simulink model "PID2"  (R2022b)
settings: Solver=VariableStepAuto  StartTime=0.0  StopTime=20  RelTol=1e-3
values from neighbouring files (symbols this model uses):
  g = 9.8    [config.m]
  Jx = 2*Mc*R^2/5 + 2*m*l^2    (= 0.0448)    [config.m]
  Jy = 2*Mc*R^2/5 + 2*m*l^2    (= 0.0448)    [config.m]
  Jz = 2*Mc*R^2/5 + 4*m*l^2    (= 0.0808)    [config.m]
  Kd_pitch = 15    [config.m]
  Kd_roll = 15    [config.m]
  Kd_yaw = 15    [config.m]
  Kd_z = 15    [config.m]
  Ki_pitch = 1    [config.m]
  Ki_roll = 1    [config.m]
  Ki_yaw = 1    [config.m]
  Ki_z = 10    [config.m]
  Kp_pitch = 80    [config.m]
  Kp_roll = 80    [config.m]
  Kp_yaw = 80    [config.m]
  Kp_z = 80    [config.m]
  M = Mc + 4*m    (= 3)    [config.m]
settings Model: Creator=cxk  LastModifiedBy=cxk

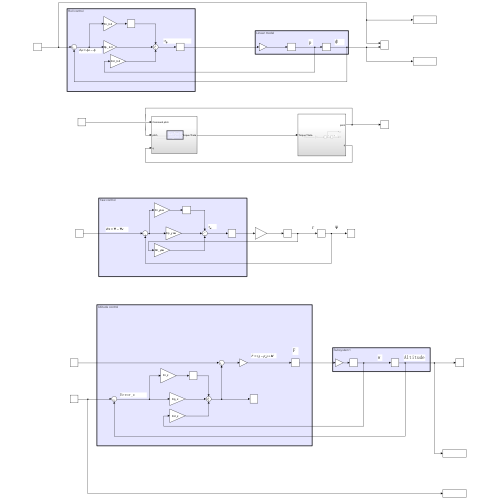
[thumbnail: Simulink's stored preview of the top-level diagram]
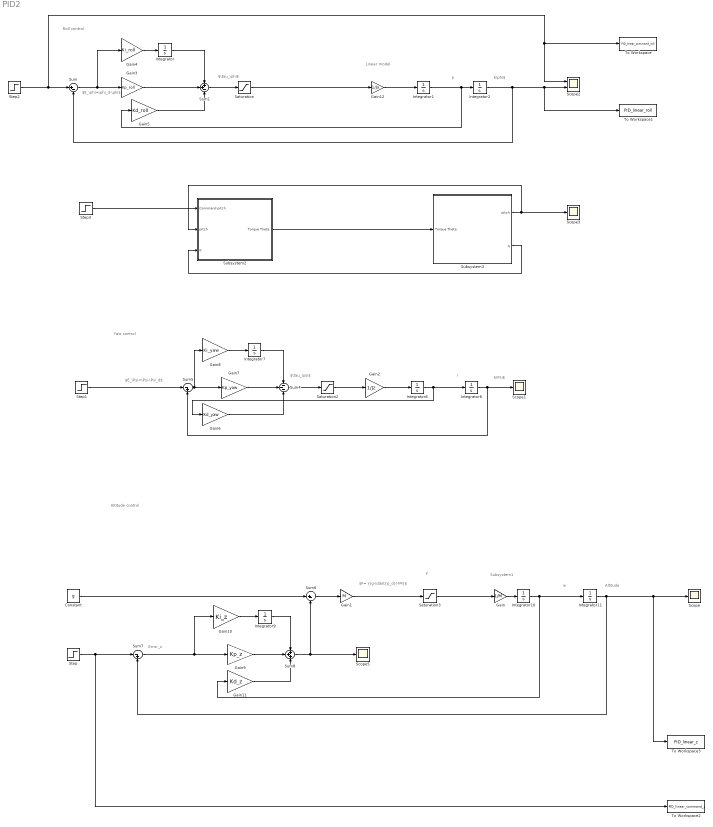
== system PID2 ==
  note: Linear model
  note: Altitude control
  note: Altitude
  note: Error_z
  note: $F= {(g-\ddot{p_d})*M}$
  note: Subsystem1
  note: w
  note: F
  note: $\tau_\psi$
  note: Yaw control
  note: $\Psi$
  note: $E_\Psi=\Psi-\Psi_d$
  note: r
  note: $\tau_\phi$
  note: Roll control
  note: $E_\phi=\phi_d-\phi$
  note: p
  note: $\phi$
  Constant : Constant  Value=g
  Gain : Gain  Gain=1/M
  Gain1 : Gain  Gain=M
  Gain10 : Gain  Gain=Ki_z
  Gain11 : Gain  Gain=Kd_z
  Gain12 : Gain  Gain=1/Jx
  Gain2 : Gain  Gain=1/Jz
  Gain3 : Gain  Gain=Kp_roll
  Gain4 : Gain  Gain=Ki_roll
  Gain5 : Gain  Gain=Kd_roll
  Gain6 : Gain  Gain=Kd_yaw
  Gain7 : Gain  Gain=Kp_yaw
  Gain8 : Gain  Gain=Ki_yaw
  Gain9 : Gain  Gain=Kp_z
  Integrator{,1..2,6..11} (9 alike) : Integrator
  Saturation : Saturate  UpperLimit=100  LowerLimit=-100
  Saturation2 : Saturate  UpperLimit=100  LowerLimit=-100
  Saturation3 : Saturate  UpperLimit=g*M*10  LowerLimit=-2.97*M*10
  Scope{,1,3,5} (4 alike) : Scope
  Scope2 : Scope  NumInputPorts=2
  Step : Step  After=-3  SampleTime=0
  Step1 : Step  SampleTime=0
  Step2 : Step  After=0.68  SampleTime=0
  Step3 : Step  After=0.68  SampleTime=0
  Subsystem2 : Subsystem
  Subsystem3 : Subsystem
  Sum : Sum  Inputs=|+-
  Sum1 : Sum  Inputs=++-
  Sum4 : Sum  Inputs=---
  Sum5 : Sum  Inputs=|-+
  Sum6 : Sum  Inputs=|+-
  Sum7 : Sum  Inputs=|-+
  Sum8 : Sum  Inputs=+++
  To Workspace : ToWorkspace  VariableName=PID_linear_command_roll  SaveFormat=Timeseries  SampleTime=-1
  To Workspace1 : ToWorkspace  VariableName=PID_linear_roll  SaveFormat=Timeseries  SampleTime=-1
  To Workspace2 : ToWorkspace  VariableName=PID_linear_command_z  SaveFormat=Timeseries  SampleTime=-1
  To Workspace3 : ToWorkspace  VariableName=PID_linear_z  SaveFormat=Timeseries  SampleTime=-1
  wires:
  Step/1 -> To Workspace2/1, Sum7/1
  Constant/1 -> Sum6/1
  Integrator11/1 -> Sum7/2, To Workspace3/1, Scope/1
  Saturation3/1 -> Gain/1
  Gain9/1 -> Sum8/2
  Gain1/1 -> Saturation3/1
  Integrator10/1 -> Integrator11/1, Gain11/1
  Gain/1 -> Integrator10/1
  Sum7/1 -> Gain10/1, Gain9/1
  Gain11/1 -> Sum8/3
  Sum8/1 -> Scope5/1, Sum6/2
  Gain10/1 -> Integrator9/1
  Integrator9/1 -> Sum8/1
  Sum6/1 -> Gain1/1
  Sum5/1 -> Gain8/1, Gain7/1
  Gain6/1 -> Sum4/3
  Integrator8/1 -> Integrator6/1, Gain6/1
  Gain2/1 -> Integrator8/1
  Saturation2/1 -> Gain2/1
  Gain8/1 -> Integrator7/1
  Step1/1 -> Sum5/1
  Integrator6/1 -> Scope1/1, Sum5/2
  Integrator7/1 -> Sum4/1
  Gain7/1 -> Sum4/2
  Sum4/1 -> Saturation2/1
  Subsystem3/1(pitch) -> Scope3/1, Subsystem2/2(pitch)
  Subsystem3/2(q) -> Subsystem2/3(q)
  Subsystem2/1(Torque Theta) -> Subsystem3/1(Torque Theta)
  Step3/1 -> Subsystem2/1(Command pitch)
  Sum/1 -> Gain4/1, Gain3/1
  Integrator/1 -> Sum1/1
  Step2/1 -> To Workspace/1, Scope2/1, Sum/1
  Integrator2/1 -> Sum/2, To Workspace1/1, Scope2/2
  Gain3/1 -> Sum1/2
  Gain5/1 -> Sum1/3
  Sum1/1 -> Saturation/1
  Gain4/1 -> Integrator/1
  Integrator1/1 -> Gain5/1, Integrator2/1
  Saturation/1 -> Gain12/1
  Gain12/1 -> Integrator1/1

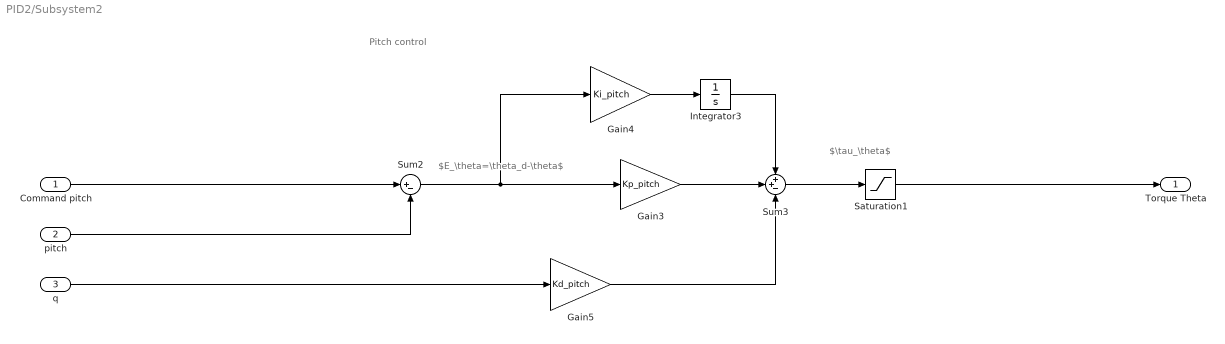
== system PID2/Subsystem2 ==
  note: Pitch control
  note: $\tau_\theta$
  note: $E_\theta=\theta_d-\theta$
  Command pitch : Inport
  pitch : Inport  Port=2
  q : Inport  Port=3
  Gain3 : Gain  Gain=Kp_pitch
  Gain4 : Gain  Gain=Ki_pitch
  Gain5 : Gain  Gain=Kd_pitch
  Integrator3 : Integrator
  Saturation1 : Saturate  UpperLimit=100  LowerLimit=-100
  Sum2 : Sum  Inputs=|+-
  Sum3 : Sum  Inputs=++-
  Torque Theta : Outport
  wires:
  Gain3/1 -> Sum3/2
  Integrator3/1 -> Sum3/1
  Sum2/1 -> Gain4/1, Gain3/1
  Sum3/1 -> Saturation1/1
  Gain5/1 -> Sum3/3
  Command pitch/1 -> Sum2/1
  Gain4/1 -> Integrator3/1
  Saturation1/1 -> Torque Theta/1
  pitch/1 -> Sum2/2
  q/1 -> Gain5/1

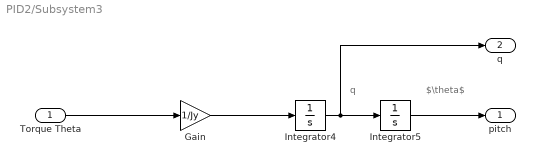
== system PID2/Subsystem3 ==
  note: q
  note: $\theta$
  Torque Theta : Inport
  Gain : Gain  Gain=1/Jy
  Integrator4 : Integrator
  Integrator5 : Integrator
  pitch : Outport
  q : Outport  Port=2
  wires:
  Integrator4/1 -> q/1, Integrator5/1
  Integrator5/1 -> pitch/1
  Torque Theta/1 -> Gain/1
  Gain/1 -> Integrator4/1
